simulink model "FINAL_1"  (R2014a)
settings: Solver=ode45  StartTime=0.0  StopTime=10.0  RelTol=1e-3
libraries: dspsrcs4 x1
settings Model: Creator=mostafa  LastModifiedBy=mostafa

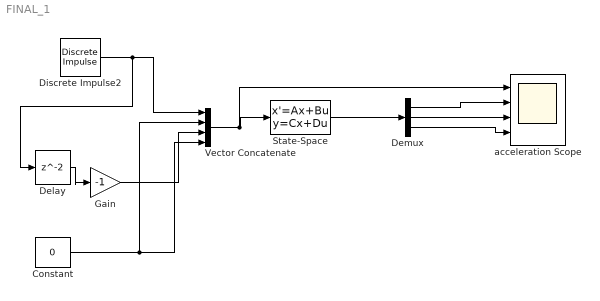
== system FINAL_1 ==
  Constant : Constant  Value=0
  Delay : Delay  InitialCondition=0
  Demux : Demux  Outputs=3
  Discrete Impulse2 : dspsrcs4/Discrete  Impulse  Delay=0  SampleTime=1  FrameSample=1  dataType=double  isSigned=on  wordLen=16  udDataType=sfix(16)  fracBitsMode=Best precision  numFracBits=15  OutDataTypeStr=double  LastOutDataTypeStr=double
  Gain : Gain  Gain=-1
  State-Space : StateSpace  A=[0 0 0;0 0 0;0 0 0 ]  B=[0 -0.05 0 0.05; -0.05 0 -.05 0;.5 -.5 .5 -.5]  C=[1 0 0;0 1 0;0 0 1]  D=[0 0 0 0;0 0 0 0;0 0 0 0 ]  X0=0
  Vector Concatenate : Concatenate  NumInputs=4
  "acceleration Scope " : Scope  NumInputPorts=4
      settings: ShowLegends=on  TimeRange=20  YMin=-10~-1.5~-0.5~-5  YMax=5~0.5~1.5~5
  wires:
  Demux/1 -> "acceleration Scope "/2
  Demux/2 -> "acceleration Scope "/3
  Demux/3 -> "acceleration Scope "/4
  State-Space/1 -> Demux/1
  Vector Concatenate/1 -> "acceleration Scope "/1, State-Space/1
  Discrete Impulse2/1 -> Delay/1, Vector Concatenate/1
  Delay/1 -> Gain/1
  Constant/1 -> Vector Concatenate/2, Vector Concatenate/4
  Gain/1 -> Vector Concatenate/3
